simulink model "Dc_Motor_Position_Crtl"  (R2020b)
settings: Solver=VariableStepAuto  StartTime=0.0  StopTime=10.0  RelTol=1e-3
values from neighbouring files (symbols this model uses):
  b = 3.5077E-6    (= 3.5077e-06)    [dc_motor_position_crtl.m]    (also in dc_motor_position_crtl_tuning.m)
  J = 3.2284E-6    (= 3.2284e-06)    [dc_motor_position_crtl.m]    (also in dc_motor_position_crtl_tuning.m)
  Kb = 0.0274    [dc_motor_position_crtl.m]    (also in dc_motor_position_crtl_tuning.m)
  Kt = 0.0274    [dc_motor_position_crtl.m]    (also in dc_motor_position_crtl_tuning.m)
  L = 2.75E-6    (= 2.75e-06)    [dc_motor_position_crtl.m]    (also in dc_motor_position_crtl_tuning.m)
  R = 4    [dc_motor_position_crtl.m]    (also in dc_motor_position_crtl_tuning.m)
  V = 1    [dc_motor_position_crtl.m]    (also in dc_motor_position_crtl_tuning.m)
settings Model: Creator=Raihan mahmud  LastModifiedBy=Raihan mahmud

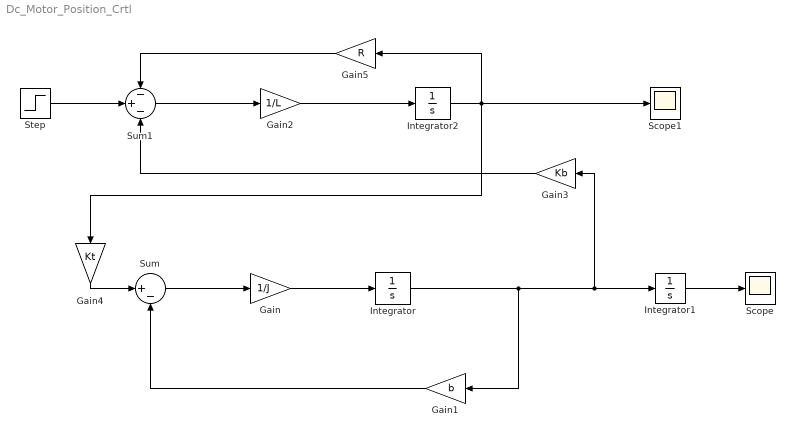
== system Dc_Motor_Position_Crtl ==
  Gain : Gain  Gain=1/J
  Gain1 : Gain  Gain=b
  Gain2 : Gain  Gain=1/L
  Gain3 : Gain  Gain=Kb
  Gain4 : Gain  Gain=Kt
  Gain5 : Gain  Gain=R
  Integrator : Integrator
  Integrator1 : Integrator
  Integrator2 : Integrator
  Scope : Scope
  Scope1 : Scope
  Step : Step  After=V  SampleTime=0
  Sum : Sum  Inputs=|+-
  Sum1 : Sum  Inputs=-+-
  wires:
  Gain/1 -> Integrator/1
  Sum/1 -> Gain/1
  Integrator/1 -> Gain3/1, Integrator1/1, Gain1/1
  Gain1/1 -> Sum/2
  Integrator1/1 -> Scope/1
  Step/1 -> Sum1/2
  Gain3/1 -> Sum1/3
  Sum1/1 -> Gain2/1
  Gain2/1 -> Integrator2/1
  Integrator2/1 -> Gain5/1, Scope1/1, Gain4/1
  Gain4/1 -> Sum/1
  Gain5/1 -> Sum1/1
